simulink model "hop_zero_ground"  (R2019a)
settings: Solver=VariableStepAuto  StartTime=0.0  StopTime=tc  RelTol=1e-3
values from neighbouring files (symbols this model uses):
  g = -9.81    [MMR.m]    (also in MMR_alfa0.m; MMR_alone.m; MMR_hop_zero.m = 9.81)
  k = 2000.0    (= 2000)    [MMR.m]    (also in MMR_alfa0.m = 22500; MMR_alone.m; MMR_hop_zero.m = 8515.125)
  M = 15    [MMR.m]    (also in MMR_alfa0.m; MMR_alone.m; MMR_hop_zero.m)
  m = 3    [MMR.m]    (also in MMR_alfa0.m; MMR_alone.m; MMR_hop_zero.m)
  vy0 = vyair( length(vyair) )    [MMR.m]    (also in MMR_alfa0.m = -0.7; MMR_alone.m; MMR_hop_zero.m = -0.613125)
  y0 = Lkf * cos(alfa0 - beta0)    [MMR.m]    (also in MMR_alfa0.m = 0.28; MMR_alone.m; MMR_hop_zero.m = 0.56)
settings Model: Creator=Jesus  LastModifiedBy=Jesus

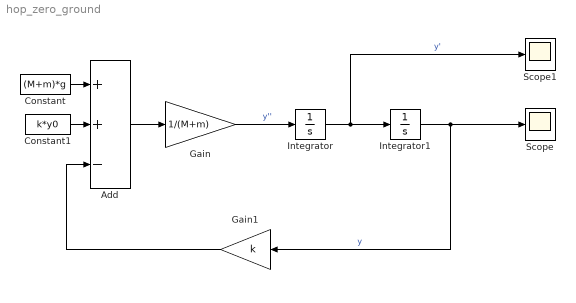
== system hop_zero_ground ==
  Add : Sum  Inputs=++-
  Constant : Constant  Value=(M+m)*g
  Constant1 : Constant  Value=k*y0
  Gain : Gain  Gain=1/(M+m)
  Gain1 : Gain  Gain=k
  Integrator : Integrator  InitialCondition=vy0
  Integrator1 : Integrator  InitialCondition=y0
  Scope : Scope
  Scope1 : Scope
  wires:
  Add/1 -> Gain/1
  Constant/1 -> Add/1
  Constant1/1 -> Add/2
  Gain/1 -> Integrator/1  "y''"
  Integrator/1 -> Scope1/1, Integrator1/1  "y'"
  Integrator1/1 -> Gain1/1, Scope/1  "y"
  Gain1/1 -> Add/3
